simulink model "sim_linear_control_debug"  (R2018a)
settings: Solver=ode1  StartTime=0.0  StopTime=1  FixedStep=0.002  RelTol=1e-3
settings Model: Creator=E183308  LastModifiedBy=E183308

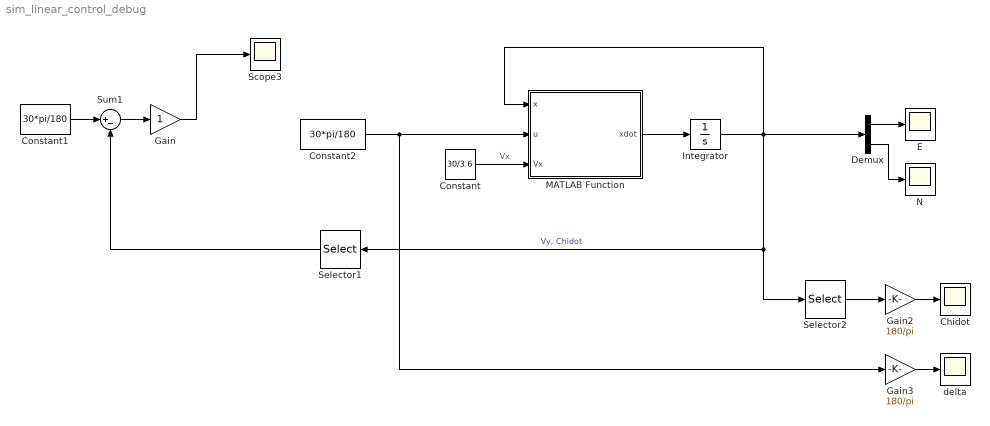
== system sim_linear_control_debug ==
  Chidot : Scope
  Constant : Constant  Value=30/3.6
  Constant1 : Constant  Value=30*pi/180
  Constant2 : Constant  Value=30*pi/180
  Demux : Demux  Outputs=2
  E : Scope
  Gain : Gain
  Gain2 : Gain  Gain=180/pi
  Gain3 : Gain  Gain=180/pi
  Integrator : Integrator  InitialCondition=[0;0]
  MATLAB Function : MATLAB Function  TreatAsAtomicUnit=on
  N : Scope
  Scope3 : Scope
  Selector1 : Selector  InputPortWidth=2  IndexOptions=Index vector (dialog)  Indices=2  OutputSizes=1
  Selector2 : Selector  InputPortWidth=2  IndexOptions=Index vector (dialog)  Indices=2  OutputSizes=1
  Sum1 : Sum  Inputs=|+-
  delta : Scope
  wires:
  Sum1/1 -> Gain/1
  Selector1/1 -> Sum1/2
  MATLAB Function/1(xdot) -> Integrator/1
  Gain/1 -> Scope3/1
  Integrator/1 -> Demux/1, Selector2/1, Selector1/1, MATLAB Function/1(x)  "Vy, Chidot"
  Constant2/1 -> Gain3/1, MATLAB Function/2(u)
  Constant1/1 -> Sum1/1
  Gain2/1 -> Chidot/1
  Selector2/1 -> Gain2/1
  Gain3/1 -> delta/1
  Constant/1 -> MATLAB Function/3(Vx)  "Vx"
  Demux/2 -> N/1
  Demux/1 -> E/1

== matlab function sim_linear_control_debug/MATLAB Function ==
  data: x input; u input; xdot output; Vx input
function xdot = dynamic_lin(x,u,Vx)

% sports sedan

m = 1724; % kg
Iz = 3400; % kg/m^2
a = 1.35; % m
b = 1.15; % m
Cf = 12*1e4; % N/rad
Cr = 175*1e3; % N/rad
mu = 0.5225;

% x = [vy Chidot], u = delta

A = [-(Cf+Cr)/m  -(a*Cf-b*Cr)/(m*Vx)-Vx; 
    -(a*Cf-b*Cr)/Iz -(a^2*Cf-b^2*Cr)/(Iz*Vx)];

B = [Cf/m; a*Cf/Iz];

xdot = A*x + B*u;
